simulink model "AGC"  (R2022a)
settings: Solver=VariableStepAuto  StartTime=0.0  StopTime=6  RelTol=1e-3
values from neighbouring files (symbols this model uses):
  a = 0.01    [Simulink.m]
  Fixeda = fi(a,1,13,12)    [Simulink.m]
  FixedR = fi(R,0,2,0)    [Simulink.m]
  Fs = 100e2    (= 10000)    [Simulink.m]
  R = 2    [Simulink.m]
settings Model: Creator=RolePyps  LastModifiedBy=RolePyps

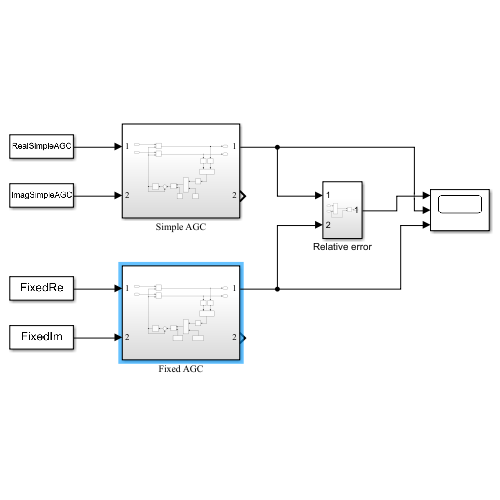
[thumbnail: Simulink's stored preview of the top-level diagram]
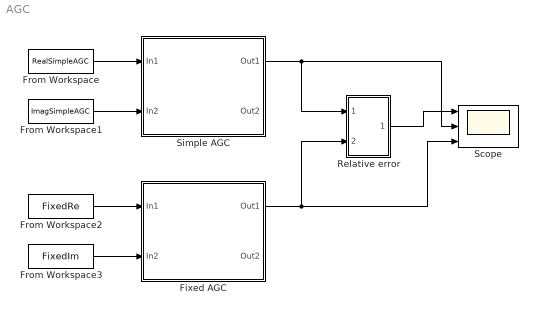
== system AGC ==
  Fixed AGC : Subsystem
  From Workspace : FromWorkspace  VariableName=RealSimpleAGC  OutDataTypeStr=double  SampleTime=1/Fs  Interpolate=off  OutputAfterFinalValue=Setting to zero
  From Workspace1 : FromWorkspace  VariableName=ImagSimpleAGC  SampleTime=1/Fs  Interpolate=off  OutputAfterFinalValue=Setting to zero
  From Workspace2 : FromWorkspace  VariableName=FixedRe  OutDataTypeStr=fixdt(1,16,14)  SampleTime=1/Fs  Interpolate=off  OutputAfterFinalValue=Setting to zero
  From Workspace3 : FromWorkspace  VariableName=FixedIm  OutDataTypeStr=fixdt(1,16,14)  SampleTime=1/Fs  Interpolate=off  OutputAfterFinalValue=Setting to zero
  Relative error : Subsystem
  Scope : Scope  NumInputPorts=3
  Simple AGC : Subsystem
  wires:
  From Workspace/1 -> Simple AGC/1(In1)
  From Workspace1/1 -> Simple AGC/2(In2)
  Simple AGC/1(Out1) -> Scope/2, Relative error/1(In1)
  Relative error/1(Out1) -> Scope/1
  From Workspace3/1 -> Fixed AGC/2(In2)
  From Workspace2/1 -> Fixed AGC/1(In1)
  Fixed AGC/1(Out1) -> Scope/3, Relative error/2(In3)

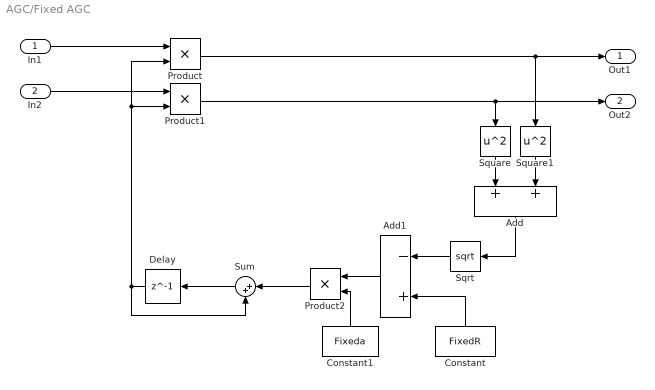
== system AGC/Fixed AGC ==
  In1 : Inport
  In2 : Inport  Port=2
  Add : Sum  AccumDataTypeStr=fixdt(1,34,22)  OutDataTypeStr=double
  Add1 : Sum  Inputs=-+  AccumDataTypeStr=fixdt(1,19,11)
  Constant : Constant  Value=FixedR
  Constant1 : Constant  Value=Fixeda
  Delay : Delay  DelayLength=1  InitialCondition=0  SampleTime=1/Fs
  Product : Product  OutDataTypeStr=fixdt(1,16,11)
  Product1 : Product  OutDataTypeStr=fixdt(1,16,11)
  Product2 : Product  OutDataTypeStr=fixdt(1,25,16)
  Sqrt : Sqrt  OutDataTypeStr=fixdt(1,18,11)
  Square : Math  Operator=square  OutDataTypeStr=fixdt(1,33,22)
  Square1 : Math  Operator=square  OutDataTypeStr=fixdt(1,33,22)
  Sum : Sum  Inputs=|++  OutDataTypeStr=fixdt(1,25,16)
  Out1 : Outport
  Out2 : Outport  Port=2
  wires:
  Square/1 -> Add/1
  Sqrt/1 -> Add1/1
  Delay/1 -> Sum/2, Product/2, Product1/2
  Product/1 -> Out1/1, Square1/1
  Add1/1 -> Product2/1
  Product1/1 -> Out2/1, Square/1
  Constant/1 -> Add1/2
  In1/1 -> Product/1
  In2/1 -> Product1/1
  Sum/1 -> Delay/1
  Product2/1 -> Sum/1
  Square1/1 -> Add/2
  Add/1 -> Sqrt/1
  Constant1/1 -> Product2/2

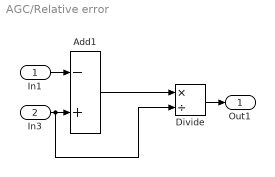
== system AGC/Relative error ==
  In1 : Inport
  In3 : Inport  Port=2
  Add1 : Sum  Inputs=-+  AccumDataTypeStr=double
  Divide : Product  Inputs=*/
  Out1 : Outport
  wires:
  Add1/1 -> Divide/1
  In3/1 -> Divide/2, Add1/2
  Divide/1 -> Out1/1
  In1/1 -> Add1/1

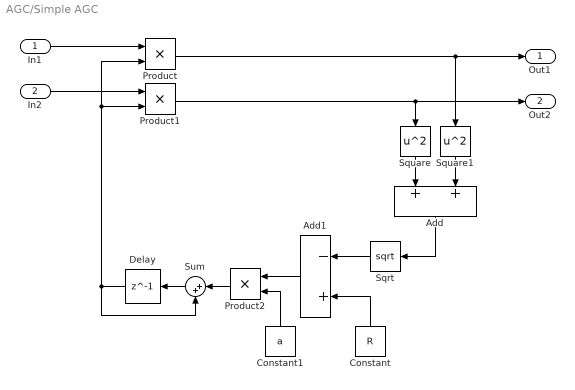
== system AGC/Simple AGC ==
  In1 : Inport
  In2 : Inport  Port=2
  Add : Sum  OutDataTypeStr=double
  Add1 : Sum  Inputs=-+  AccumDataTypeStr=double
  Constant : Constant  Value=R
  Constant1 : Constant  Value=a
  Delay : Delay  DelayLength=1  InitialCondition=0
  Product : Product  OutDataTypeStr=double
  Product1 : Product  OutDataTypeStr=double
  Product2 : Product  OutDataTypeStr=double
  Sqrt : Sqrt  OutDataTypeStr=double
  Square : Math  Operator=square  OutDataTypeStr=double
  Square1 : Math  Operator=square  OutDataTypeStr=double
  Sum : Sum  Inputs=|++  AccumDataTypeStr=double
  Out1 : Outport
  Out2 : Outport  Port=2
  wires:
  Square/1 -> Add/1
  Sqrt/1 -> Add1/1
  Delay/1 -> Sum/2, Product1/2, Product/2
  Product/1 -> Out1/1, Square1/1
  Add1/1 -> Product2/1
  Product1/1 -> Out2/1, Square/1
  Constant/1 -> Add1/2
  In1/1 -> Product/1
  In2/1 -> Product1/1
  Sum/1 -> Delay/1
  Product2/1 -> Sum/1
  Square1/1 -> Add/2
  Add/1 -> Sqrt/1
  Constant1/1 -> Product2/2
